simulink model "untitled2"  (R2018b)
settings: Solver=VariableStepAuto  StartTime=0.0  StopTime=20.0  RelTol=1e-3
settings Model: Creator=zhele  LastModifiedBy=zhele

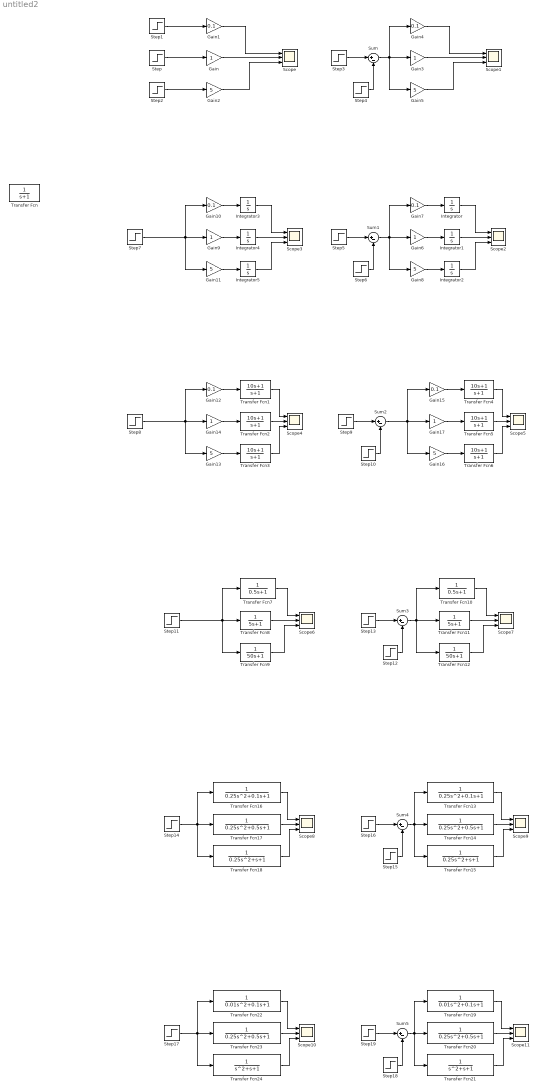
== system untitled2 ==
  Gain{,3,6,9,14,17} (6 alike) : Gain
  Gain{1,4,7,10,12,15} (6 alike) : Gain  Gain=0.1
  Gain{2,5,8,11,13,16} (6 alike) : Gain  Gain=5
  Integrator{,1..5} (6 alike) : Integrator
  Scope{,1..11} (12 alike) : Scope  NumInputPorts=3
  Step{,1..3,5,7..9,11,13..14,16..17,19} (14 alike) : Step  After=10  SampleTime=0
  Step{4,6,10,12,15,18} (6 alike) : Step  Time=1.2  After=10  SampleTime=0
  Sum{,1..5} (6 alike) : Sum  Inputs=|+-
  Transfer Fcn : TransferFcn  Denominator=[1 1]
  Transfer Fcn{1..6} (6 alike) : TransferFcn  Numerator=[10 1]  Denominator=[1 1]
  Transfer Fcn10 : TransferFcn  Denominator=[0.5 1]
  Transfer Fcn11 : TransferFcn  Denominator=[5 1]
  Transfer Fcn12 : TransferFcn  Denominator=[50 1]
  Transfer Fcn13 : TransferFcn  Denominator=[0.25 0.1 1]
  Transfer Fcn{14,17,20,23} (4 alike) : TransferFcn  Denominator=[0.25 0.5 1]
  Transfer Fcn15 : TransferFcn  Denominator=[0.25 1 1]
  Transfer Fcn16 : TransferFcn  Denominator=[0.25 0.1 1]
  Transfer Fcn18 : TransferFcn  Denominator=[0.25 1 1]
  Transfer Fcn19 : TransferFcn  Denominator=[0.01 0.1 1]
  Transfer Fcn21 : TransferFcn  Denominator=[1 1 1]
  Transfer Fcn22 : TransferFcn  Denominator=[0.01 0.1 1]
  Transfer Fcn24 : TransferFcn  Denominator=[1 1 1]
  Transfer Fcn7 : TransferFcn  Denominator=[0.5 1]
  Transfer Fcn8 : TransferFcn  Denominator=[5 1]
  Transfer Fcn9 : TransferFcn  Denominator=[50 1]
  wires:
  Step/1 -> Gain/1
  Gain/1 -> Scope/2
  Gain1/1 -> Scope/1
  Step1/1 -> Gain1/1
  Step2/1 -> Gain2/1
  Gain2/1 -> Scope/3
  Step4/1 -> Sum/2
  Step3/1 -> Sum/1
  Gain5/1 -> Scope1/3
  Gain4/1 -> Scope1/1
  Gain3/1 -> Scope1/2
  Sum/1 -> Gain5/1, Gain4/1, Gain3/1
  Step5/1 -> Sum1/1
  Step6/1 -> Sum1/2
  Sum1/1 -> Gain8/1, Gain7/1, Gain6/1
  Gain7/1 -> Integrator/1
  Integrator/1 -> Scope2/1
  Gain6/1 -> Integrator1/1
  Integrator1/1 -> Scope2/2
  Gain8/1 -> Integrator2/1
  Integrator2/1 -> Scope2/3
  Gain11/1 -> Integrator5/1
  Integrator5/1 -> Scope3/3
  Gain9/1 -> Integrator4/1
  Integrator4/1 -> Scope3/2
  Gain10/1 -> Integrator3/1
  Integrator3/1 -> Scope3/1
  Step7/1 -> Gain11/1, Gain10/1, Gain9/1
  Gain12/1 -> Transfer Fcn1/1
  Gain14/1 -> Transfer Fcn2/1
  Gain13/1 -> Transfer Fcn3/1
  Step8/1 -> Gain13/1, Gain12/1, Gain14/1
  Transfer Fcn1/1 -> Scope4/1
  Transfer Fcn2/1 -> Scope4/2
  Transfer Fcn3/1 -> Scope4/3
  Transfer Fcn6/1 -> Scope5/3
  Transfer Fcn5/1 -> Scope5/2
  Gain17/1 -> Transfer Fcn5/1
  Sum2/1 -> Gain15/1, Gain16/1, Gain17/1
  Gain16/1 -> Transfer Fcn6/1
  Transfer Fcn4/1 -> Scope5/1
  Gain15/1 -> Transfer Fcn4/1
  Step9/1 -> Sum2/1
  Step10/1 -> Sum2/2
  Step11/1 -> Transfer Fcn9/1, Transfer Fcn8/1, Transfer Fcn7/1
  Transfer Fcn7/1 -> Scope6/1
  Transfer Fcn8/1 -> Scope6/2
  Transfer Fcn9/1 -> Scope6/3
  Step13/1 -> Sum3/1
  Step12/1 -> Sum3/2
  Transfer Fcn11/1 -> Scope7/2
  Transfer Fcn12/1 -> Scope7/3
  Transfer Fcn10/1 -> Scope7/1
  Sum3/1 -> Transfer Fcn12/1, Transfer Fcn10/1, Transfer Fcn11/1
  Step14/1 -> Transfer Fcn17/1, Transfer Fcn16/1, Transfer Fcn18/1
  Step15/1 -> Sum4/2
  Step16/1 -> Sum4/1
  Transfer Fcn16/1 -> Scope8/1
  Transfer Fcn17/1 -> Scope8/2
  Transfer Fcn18/1 -> Scope8/3
  Transfer Fcn13/1 -> Scope9/1
  Transfer Fcn15/1 -> Scope9/3
  Sum4/1 -> Transfer Fcn15/1, Transfer Fcn13/1, Transfer Fcn14/1
  Transfer Fcn14/1 -> Scope9/2
  Transfer Fcn23/1 -> Scope10/2
  Step17/1 -> Transfer Fcn23/1, Transfer Fcn22/1, Transfer Fcn24/1
  Transfer Fcn20/1 -> Scope11/2
  Transfer Fcn19/1 -> Scope11/1
  Transfer Fcn24/1 -> Scope10/3
  Sum5/1 -> Transfer Fcn20/1, Transfer Fcn21/1, Transfer Fcn19/1
  Step18/1 -> Sum5/2
  Transfer Fcn21/1 -> Scope11/3
  Step19/1 -> Sum5/1
  Transfer Fcn22/1 -> Scope10/1
